simulink model "testjtraj"  (R2014b)
settings: Solver=ode3  StartTime=0.0  StopTime=10.0  FixedStep=0.01  RelTol=1e-3
InitFcn:
  | Tm = 0.01;
  | 
  | tm = 0.01;
  | tj = 3;
  | tt = 10;
  | t1 = 0;
  | t2 = 5;
  | q0 = 0;
  | q1 = -50;
  | q2 = 50;
  | 
  | T = 0:tm:tj;
  | [qd1,qd1p,qd1pp] = jtraj(q0,q1,T);
  | [qd2,qd2p,qd2pp] = jtraj(q1,q2,T);
  | 
  | qds0 = ones(t1/tm,1)*q0;
  | qds1 = ones((t2-t1-tj)/tm,1)*q1;
  | qds2 = ones((tt-t2-tj)/tm,1)*q2;
  | 
  | qd = [qds0;qd1;qds1;qd2;qds2];
  | qdp = [qds0*0;qd1p;qds1*0;qd2p;qds2*0];
  | qdpp = [qds0*0;qd1pp;qds1*0;qd2pp;qds2*0];
  | tt = (0:tm:tt)';
  | qd = qd(1:length(tt));
  | qdp = qdp(1:length(tt));
  | qdpp = qdpp(1:length(tt));
  | 
  | %subplot(3,1,1), plot(tt,qd)
  | %subplot(3,1,2), plot(tt,qdp)
  | %subplot(3,1,3), plot(tt,qdpp)
  | 
  | spq.time = tt;
  | spq.signals.values = [qd qdp qdpp];
  | 
  | 
  | 
  | %tss = 1.5;
  | fi = 0.707;
  | 
  | k = 360/60;
  | km = 10;
  | tm = 0.5;
  | 
  | tv = tm;
  | %wn = 4/(fi*tss);
  | wn = 2*pi*5/7; % wn/2pi < Fc/10 (Fc: Fc de los filtros de la medición)
  | %wn = 2*pi*5;
  | kp = wn/(2*fi*k);
  | kv = 2*fi*wn*tv/km;
  | 
  | KA = tv/(kp*kv*km*k);
  | KV = 1/(kp*k);
undefined symbols (not defined in the file or in its folder): A, B, Humusoft, MF624
libraries: rtwinlib x3
settings Model: SimulationMode=external  ExtModeTrigDuration=1000000  Creator=Servo  LastModifiedBy=Servo
settings HardwareCC: ProdIntDivRoundTo=Zero  ProdEndianess=LittleEndian  ProdHWDeviceType=Generic->32-bit x86 compatible
settings RTWCC: SystemTargetFile=rtwin.tlc  TemplateMakefile=rtwin.tmf  Description=Real-Time Windows Target  ProcessScript=rtwin_make_rtw_hook  RTWCompilerOptimization=On
settings CodeAppCC: MaxIdLength=95
settings RTWinTargetCC: TargetLibSuffix=_rtwin.lib  TargetPreCompLibLocation=C:\Program Files\MATLAB\R2014b\toolbox\rtw\targets\rtwin\lib\win64

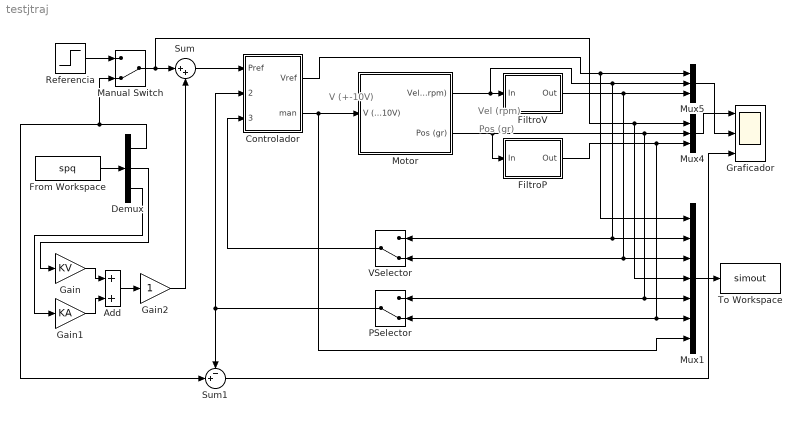
== system testjtraj ==
  note: Vel
      | (rpm)
  note: Pos
      | (gr)
  note: V (+-10V)
  Add : Sum
  Controlador : Subsystem  mask{T=0.01, Pp=kp, Ip=0, Kbp=0, Dp=0, Fcdp=5, Pv=kv, Iv=kv/tv, Kbv=1, Dv=0, Fcdv=5}
      mask prompts: T "Período de muestreo"; Kbp "Kbp (anti windup)"; Fcdp "Fcdp (Hz)"; Kbv "Kbv (anti windup)"; Fcdv "Fcdv (Hz)"
      mask init:
      | Np = 2*pi*Fcdp;
      | Nv = 2*pi*Fcdv;
  Demux : Demux  Outputs=3
  FiltroP : Subsystem  mask{N=2, Fc=5, Fm=1/0.01}
      mask prompts: N "Orden del filtro (Butterworth)"; Fc "Frecuencia de corte (Fc<Fm/2)"; Fm "Frecuencia de muestreo"
      mask init:
      | Fn = Fm/2;   % Frecuencia de Nyquist
      | [B,A] = butter(N,Fc/Fn);
  FiltroV : Subsystem  mask{N=2, Fc=5, Fm=1/0.01}
      mask prompts: N "Orden del filtro (Butterworth)"; Fc "Frecuencia de corte (Fc<Fm/2)"; Fm "Frecuencia de muestreo"
      mask init:
      | Fn = Fm/2;   % Frecuencia de Nyquist
      | [B,A] = butter(N,Fc/Fn);
  From Workspace : FromWorkspace  VariableName=spq  SampleTime=0
  Gain : Gain  Gain=KV
  Gain1 : Gain  Gain=KA
  Gain2 : Gain
  Graficador : Scope  NumInputPorts=3
      settings: TimeRange=10  YMin=-100~-100~-10  YMax=100~100~10  SampleTime=Tm
  Manual Switch : ManualSwitch  CurrentSetting=0
  Motor : Subsystem
  Mux1 : Mux  Inputs=7
  Mux4 : Mux  Inputs=3
  Mux5 : Mux  Inputs=3
  PSelector : ManualSwitch  CurrentSetting=0
  Referencia : Step  Time=5  Before=-50  After=50  SampleTime=0.01
  Sum : Sum  Inputs=|++
  Sum1 : Sum  Inputs=-+|
  To Workspace : ToWorkspace  VariableName=simout  SaveFormat=Structure With Time  SampleTime=Tm
  VSelector : ManualSwitch  CurrentSetting=0
  wires:
  Motor/2(Pos (gr)) -> Mux1/5, PSelector/1, Mux4/2, FiltroP/1(In)
  Referencia/1 -> Manual Switch/1
  FiltroP/1(Out) -> Mux1/6, PSelector/2, Mux4/3
  PSelector/1 -> Sum1/1, Controlador/2(Pmed)
  Controlador/2(man) -> Motor/1(V (+-10V)), Mux1/7
  Motor/1(Vel (rpm)) -> FiltroV/1(In), Mux5/2, VSelector/1, Mux1/2
  FiltroV/1(Out) -> Mux5/3, Mux1/3, VSelector/2
  Controlador/1(Vref) -> Mux5/1, Mux1/1
  VSelector/1 -> Controlador/3(Vmed)
  Mux1/1 -> To Workspace/1
  Mux4/1 -> Graficador/1
  Mux5/1 -> Graficador/2
  From Workspace/1 -> Demux/1
  Demux/2 -> Gain/1
  Demux/3 -> Gain1/1
  Gain/1 -> Add/1
  Gain1/1 -> Add/2
  Add/1 -> Gain2/1
  Demux/1 -> Sum1/2, Manual Switch/2
  Gain2/1 -> Sum/2
  Sum1/1 -> Graficador/3
  Manual Switch/1 -> Mux4/1, Mux1/4, Sum/1
  Sum/1 -> Controlador/1(Pref)

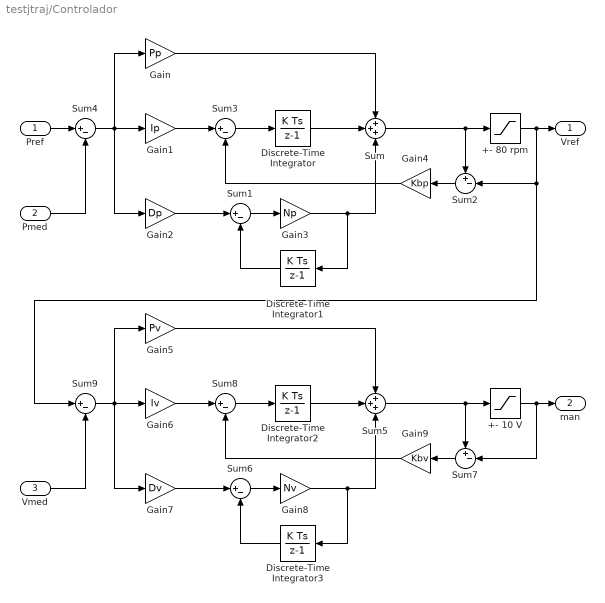
== system testjtraj/Controlador ==
  Pref : Inport
  Pmed : Inport  Port=2
  Vmed : Inport  Port=3
  +- 10 V : Saturate  UpperLimit=10  LowerLimit=-10
  +- 80 rpm : Saturate  UpperLimit=80  LowerLimit=-80
  Discrete-Time Integrator{,1..3} (4 alike) : DiscreteIntegrator  SampleTime=T
  Gain : Gain  Gain=Pp
  Gain1 : Gain  Gain=Ip
  Gain2 : Gain  Gain=Dp
  Gain3 : Gain  Gain=Np
  Gain4 : Gain  Gain=Kbp
  Gain5 : Gain  Gain=Pv
  Gain6 : Gain  Gain=Iv
  Gain7 : Gain  Gain=Dv
  Gain8 : Gain  Gain=Nv
  Gain9 : Gain  Gain=Kbv
  Sum : Sum  Inputs=+++
  Sum{1,3..4,6,8..9} (6 alike) : Sum  Inputs=|+-
  Sum2 : Sum  Inputs=+-|
  Sum5 : Sum  Inputs=+++
  Sum7 : Sum  Inputs=+-|
  Vref : Outport
  man : Outport  Port=2
  wires:
  Vmed/1 -> Sum9/2
  Sum9/1 -> Gain5/1, Gain6/1, Gain7/1
  Gain9/1 -> Sum8/2
  Gain6/1 -> Sum8/1
  Sum8/1 -> Discrete-Time Integrator2/1
  Sum7/1 -> Gain9/1
  Gain8/1 -> Sum5/3, Discrete-Time Integrator3/1
  Discrete-Time Integrator3/1 -> Sum6/2
  Gain7/1 -> Sum6/1
  Sum6/1 -> Gain8/1
  +- 80 rpm/1 -> Vref/1, Sum2/2, Sum9/1
  Discrete-Time Integrator2/1 -> Sum5/2
  Gain5/1 -> Sum5/1
  +- 10 V/1 -> Sum7/2, man/1
  Sum5/1 -> Sum7/1, +- 10 V/1
  Pmed/1 -> Sum4/2
  Sum4/1 -> Gain1/1, Gain/1, Gain2/1
  Gain4/1 -> Sum3/2
  Gain1/1 -> Sum3/1
  Sum3/1 -> Discrete-Time Integrator/1
  Sum2/1 -> Gain4/1
  Gain3/1 -> Discrete-Time Integrator1/1, Sum/3
  Discrete-Time Integrator1/1 -> Sum1/2
  Gain2/1 -> Sum1/1
  Sum1/1 -> Gain3/1
  Pref/1 -> Sum4/1
  Discrete-Time Integrator/1 -> Sum/2
  Gain/1 -> Sum/1
  Sum/1 -> +- 80 rpm/1, Sum2/1

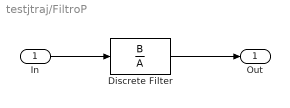
== system testjtraj/FiltroP ==
  In : Inport
  Discrete Filter : DiscreteFilter  Numerator=B  Denominator=A  SampleTime=1/Fm
  Out : Outport
  wires:
  In/1 -> Discrete Filter/1
  Discrete Filter/1 -> Out/1

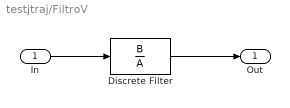
== system testjtraj/FiltroV ==
  In : Inport
  Discrete Filter : DiscreteFilter  Numerator=B  Denominator=A  SampleTime=1/Fm
  Out : Outport
  wires:
  Discrete Filter/1 -> Out/1
  In/1 -> Discrete Filter/1

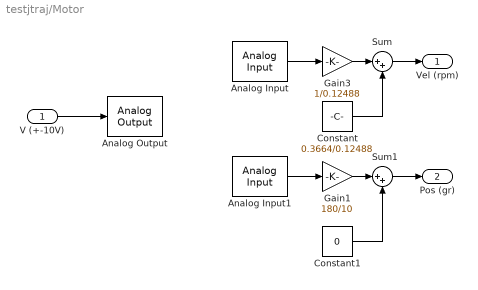
== system testjtraj/Motor ==
  V (+-10V) : Inport
  Analog Input : rtwinlib/Analog Input  SampleTime=Tm  MaxMissedTicks=10  ShowMissedTicks=off  YieldWhenWaiting=off  DrvName=Humusoft/MF624  DrvAddress=0  DrvOptions=0  Channels=1  RangeMode=1  VoltRange=1  DataType=1
      settings: AttributesFormatString=Humusoft\nMF624 [0h]
  Analog Input1 : rtwinlib/Analog Input  SampleTime=Tm  MaxMissedTicks=10  ShowMissedTicks=off  YieldWhenWaiting=off  DrvName=Humusoft/MF624  DrvAddress=0  DrvOptions=0  Channels=2  RangeMode=1  VoltRange=1  DataType=1
      settings: AttributesFormatString=Humusoft\nMF624 [0h]
  Analog Output : rtwinlib/Analog Output  SampleTime=Tm  MaxMissedTicks=10  ShowMissedTicks=off  YieldWhenWaiting=off  DrvName=Humusoft/MF624  DrvAddress=0  DrvOptions=0  Channels=1  RangeMode=1  VoltRange=1  InitialValue=0  FinalValue=0
      settings: AttributesFormatString=Humusoft\nMF624 [0h]
  Constant : Constant  Value=0.3664/0.12488
  Constant1 : Constant  Value=0
  Gain1 : Gain  Gain=180/10
  Gain3 : Gain  Gain=1/0.12488
  Sum : Sum  Inputs=|++
  Sum1 : Sum  Inputs=|++
  Vel (rpm) : Outport
  Pos (gr) : Outport  Port=2
  wires:
  Sum1/1 -> Pos (gr)/1
  Gain1/1 -> Sum1/1
  Constant1/1 -> Sum1/2
  Analog Input1/1 -> Gain1/1
  Gain3/1 -> Sum/1
  Sum/1 -> Vel (rpm)/1
  Constant/1 -> Sum/2
  Analog Input/1 -> Gain3/1
  V (+-10V)/1 -> Analog Output/1
